simulink model "Cursed"  (R2024a)
settings: Solver=VariableStepAuto  StartTime=0.0  StopTime=10.0  RelTol=1e-3
values from neighbouring files (symbols this model uses):
  mu = mM/mE    (= 0.0123053687173)    [Lab5.m]    (also in Lab8.m; chatGPT.m = 0.0121505856096)
settings Model: Creator=sgtjake2  LastModifiedBy=sgtjake2

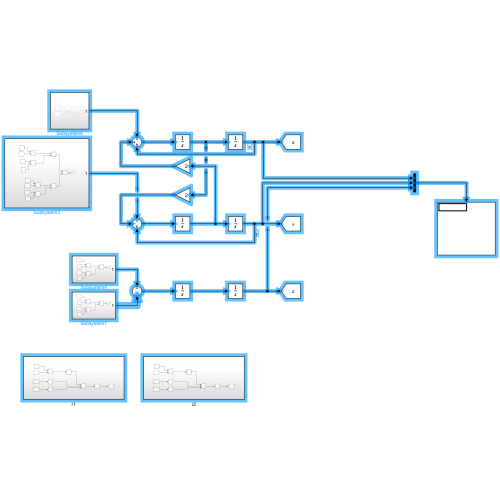
[thumbnail: Simulink's stored preview of the top-level diagram]
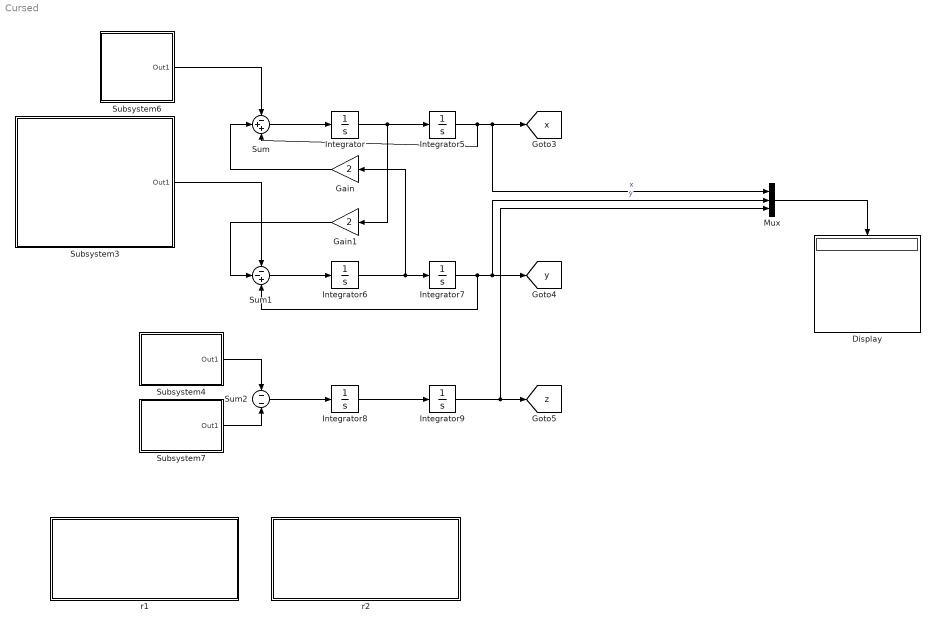
== system Cursed ==
  Display : Display
  Gain : Gain  Gain=2
  Gain1 : Gain  Gain=2
  Integrator{,5..9} (6 alike) : Integrator  InitialCondition=1
  Mux : Mux  Inputs=3
  Subsystem3 : Subsystem
  Subsystem4 : Subsystem
  Subsystem6 : Subsystem
  Subsystem7 : Subsystem
  Sum : Sum  Inputs=-++
  Sum1 : Sum  Inputs=--+
  Sum2 : Sum  Inputs=--
  r1 : Subsystem
  r2 : Subsystem
  tag scope: x=global, y=global, z=global
  wires:
  Gain1/1 -> Sum1/2
  Subsystem4/1(Out1) -> Sum2/1
  Integrator8/1 -> Integrator9/1
  Mux/1 -> Display/1
  Integrator7/1 -> Mux/2, [y], Sum1/3  "y"
  Gain/1 -> Sum/2
  Sum2/1 -> Integrator8/1
  Subsystem6/1(Out1) -> Sum/1
  Integrator9/1 -> Mux/3, [z]
  Integrator/1 -> Gain1/1, Integrator5/1
  Integrator5/1 -> Mux/1, [x], Sum/3  "x"
  Subsystem3/1(Out1) -> Sum1/1
  Integrator6/1 -> Gain/1, Integrator7/1
  Sum/1 -> Integrator/1
  Sum1/1 -> Integrator6/1
  Subsystem7/1(Out1) -> Sum2/2

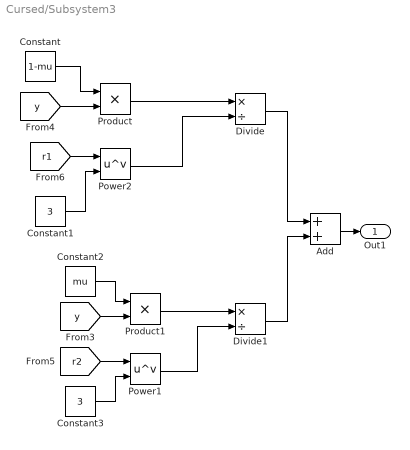
== system Cursed/Subsystem3 ==
  Add : Sum
  Constant : Constant  Value=1-mu
  Constant1 : Constant  Value=3
  Constant2 : Constant  Value=mu
  Constant3 : Constant  Value=3
  Divide : Product  Inputs=*/
  Divide1 : Product  Inputs=*/
  Power1 : Math  Operator=pow
  Power2 : Math  Operator=pow
  Product : Product
  Product1 : Product
  Out1 : Outport
  wires:
  Divide/1 -> Add/1
  Constant/1 -> Product/1
  Constant2/1 -> Product1/1
  Constant1/1 -> Power2/2
  Constant3/1 -> Power1/2
  Divide1/1 -> Add/2
  Power2/1 -> Divide/2
  Product/1 -> Divide/1
  [r1] -> Power2/1
  [y] -> Product1/2
  [r2] -> Power1/1
  Power1/1 -> Divide1/2
  Product1/1 -> Divide1/1
  [y] -> Product/2
  Add/1 -> Out1/1

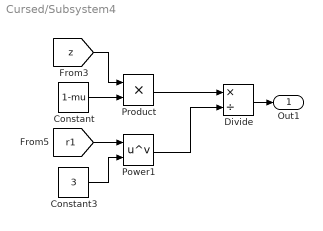
== system Cursed/Subsystem4 ==
  Constant : Constant  Value=1-mu
  Constant3 : Constant  Value=3
  Divide : Product  Inputs=*/
  Power1 : Math  Operator=pow
  Product : Product
  Out1 : Outport
  wires:
  Constant/1 -> Product/2
  Divide/1 -> Out1/1
  [z] -> Product/1
  [r1] -> Power1/1
  Power1/1 -> Divide/2
  Product/1 -> Divide/1
  Constant3/1 -> Power1/2

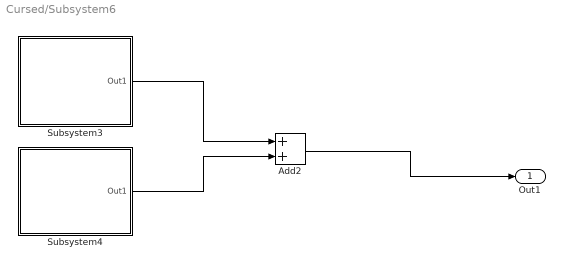
== system Cursed/Subsystem6 ==
  Add2 : Sum
  Subsystem3 : Subsystem
  Subsystem4 : Subsystem
  Out1 : Outport
  wires:
  Subsystem4/1(Out1) -> Add2/2
  Subsystem3/1(Out1) -> Add2/1
  Add2/1 -> Out1/1

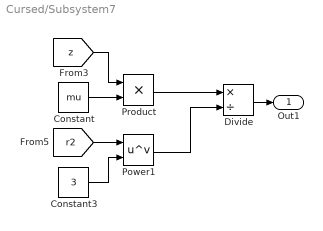
== system Cursed/Subsystem7 ==
  Constant : Constant  Value=mu
  Constant3 : Constant  Value=3
  Divide : Product  Inputs=*/
  Power1 : Math  Operator=pow
  Product : Product
  Out1 : Outport
  wires:
  Constant/1 -> Product/2
  Divide/1 -> Out1/1
  [z] -> Product/1
  [r2] -> Power1/1
  Power1/1 -> Divide/2
  Product/1 -> Divide/1
  Constant3/1 -> Power1/2

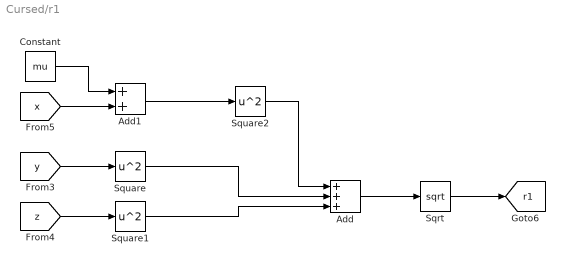
== system Cursed/r1 ==
  Add : Sum  Inputs=+++
  Add1 : Sum
  Constant : Constant  Value=mu
  Sqrt : Sqrt
  Square : Math  Operator=square
  Square1 : Math  Operator=square
  Square2 : Math  Operator=square
  tag scope: r1=global
  wires:
  Constant/1 -> Add1/1
  Square1/1 -> Add/3
  [z] -> Square1/1
  Add1/1 -> Square2/1
  [x] -> Add1/2
  [y] -> Square/1
  Sqrt/1 -> [r1]
  Add/1 -> Sqrt/1
  Square2/1 -> Add/1
  Square/1 -> Add/2

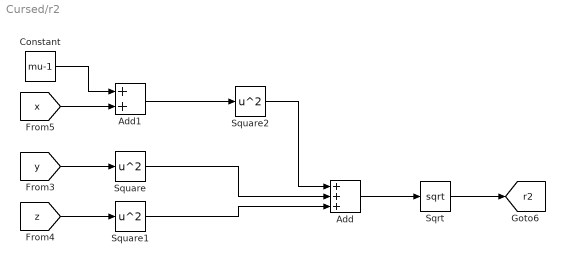
== system Cursed/r2 ==
  Add : Sum  Inputs=+++
  Add1 : Sum
  Constant : Constant  Value=mu-1
  Sqrt : Sqrt
  Square : Math  Operator=square
  Square1 : Math  Operator=square
  Square2 : Math  Operator=square
  tag scope: r2=global
  wires:
  Constant/1 -> Add1/1
  Square1/1 -> Add/3
  [z] -> Square1/1
  Add1/1 -> Square2/1
  [x] -> Add1/2
  [y] -> Square/1
  Sqrt/1 -> [r2]
  Add/1 -> Sqrt/1
  Square2/1 -> Add/1
  Square/1 -> Add/2

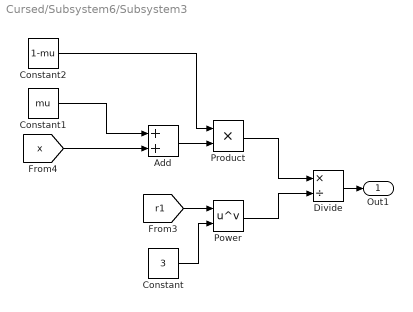
== system Cursed/Subsystem6/Subsystem3 ==
  Add : Sum
  Constant : Constant  Value=3
  Constant1 : Constant  Value=mu
  Constant2 : Constant  Value=1-mu
  Divide : Product  Inputs=*/
  Power : Math  Operator=pow
  Product : Product
  Out1 : Outport
  wires:
  Constant/1 -> Power/2
  [x] -> Add/2
  Constant1/1 -> Add/1
  Product/1 -> Divide/1
  [r1] -> Power/1
  Constant2/1 -> Product/1
  Power/1 -> Divide/2
  Add/1 -> Product/2
  Divide/1 -> Out1/1

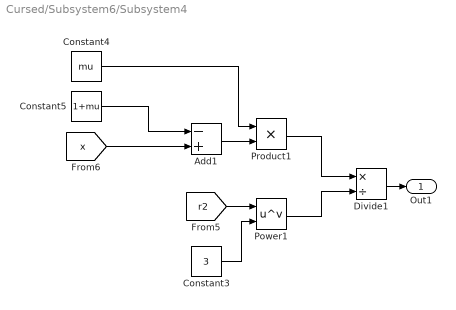
== system Cursed/Subsystem6/Subsystem4 ==
  Add1 : Sum  Inputs=-+
  Constant3 : Constant  Value=3
  Constant4 : Constant  Value=mu
  Constant5 : Constant  Value=1+mu
  Divide1 : Product  Inputs=*/
  Power1 : Math  Operator=pow
  Product1 : Product
  Out1 : Outport
  wires:
  Product1/1 -> Divide1/1
  Constant4/1 -> Product1/1
  Constant3/1 -> Power1/2
  Power1/1 -> Divide1/2
  Add1/1 -> Product1/2
  [r2] -> Power1/1
  [x] -> Add1/2
  Constant5/1 -> Add1/1
  Divide1/1 -> Out1/1
